simulink model "auditory_nerve_sim"  (R2020b)
settings: Solver=FixedStepDiscrete  StartTime=0.0  StopTime=stopTime  RelTol=1e-3
InitFcn:
  | initCallback
StopFcn:
  | stopCallback
values from neighbouring files (symbols this model uses):
  Fs = 48e3    (= 48000)    [modelparameters.m]
undefined symbols (not defined in the file or in its folder): mp
libraries: dspsrcs4 x1
settings Model: Creator=Ross  LastModifiedBy=wickh
settings DataIOCC: ReturnWorkspaceOutputs=off
settings OptimizationCC: BlockReduction=off  ConditionallyExecuteInputs=off  DefaultParameterBehavior=Inlined
settings DebuggingCC: ReadBeforeWriteMsg=DisableAll  WriteAfterWriteMsg=DisableAll  WriteAfterReadMsg=DisableAll  AlgebraicLoopMsg=error  MultiTaskDSMMsg=none  SingleTaskRateTransMsg=error  PregeneratedLibrarySubsystemCodeDiagnostic=none  ArithmeticOperatorsInVariantConditions=warning
settings HardwareCC: ProdBitPerPointer=32  ProdBitPerSizeT=32  ProdBitPerPtrDiffT=32  ProdLargestAtomicFloat=None  ProdIntDivRoundTo=Undefined  ProdEndianess=Unspecified  ProdWordSize=32  ProdHWDeviceType=ASIC/FPGA->ASIC/FPGA  TargetBitPerPointer=64  TargetBitPerSizeT=64  TargetBitPerPtrDiffT=64  TargetLongLongMode=on  TargetIntDivRoundTo=Zero  TargetEndianess=LittleEndian  TargetWordSize=64  TargetHWDeviceType=Custom Processor->MATLAB Host Computer  ProdEqTarget=off
settings ModelReferenceCC: UpdateModelReferenceTargets=IfOutOfDate
settings SFSimCC: SFSimEcho=off  SimUseLocalCustomCode=off  CustomCodeUndefinedFunction=UseInterfaceOnly
settings RTWCC: RTWUseLocalCustomCode=off

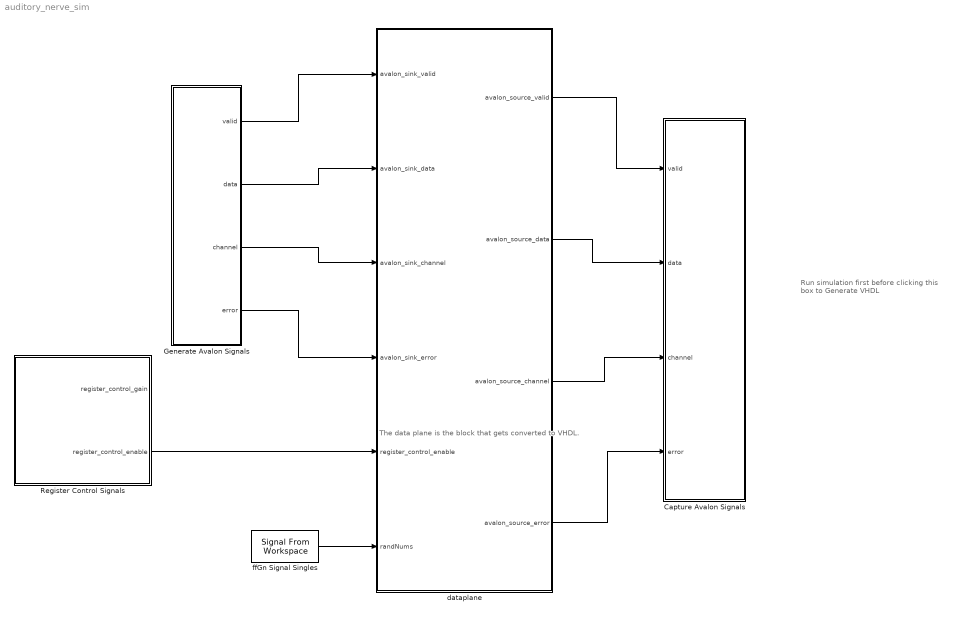
== system auditory_nerve_sim ==
  note: The data plane is the block that gets converted to VHDL.
  note: Run simulation first
      | before clicking this box to
      | Generate VHDL
  Capture Avalon Signals : Subsystem
  Generate Avalon Signals : Subsystem
  Register Control Signals : Subsystem
  dataplane : Subsystem  TreatAsAtomicUnit=on
  ffGn Signal Singles : dspsrcs4/Signal From Workspace  X=randNums  Ts=1/Fs  nsamps=1  OutputAfterFinalValue=Setting to zero  ignoreOrWarnInputAndFrameLengths=off  OutputFrames=off
  wires:
  Generate Avalon Signals/2(data) -> dataplane/2(avalon_sink_data)
  Generate Avalon Signals/1(valid) -> dataplane/1(avalon_sink_valid)
  Generate Avalon Signals/3(channel) -> dataplane/3(avalon_sink_channel)
  Generate Avalon Signals/4(error) -> dataplane/4(avalon_sink_error)
  dataplane/2(avalon_source_data) -> Capture Avalon Signals/2(data)
  dataplane/1(avalon_source_valid) -> Capture Avalon Signals/1(valid)
  dataplane/3(avalon_source_channel) -> Capture Avalon Signals/3(channel)
  dataplane/4(avalon_source_error) -> Capture Avalon Signals/4(error)
  Register Control Signals/2(register_control_enable) -> dataplane/5(register_control_enable)
  ffGn Signal Singles/1 -> dataplane/6(randNums)

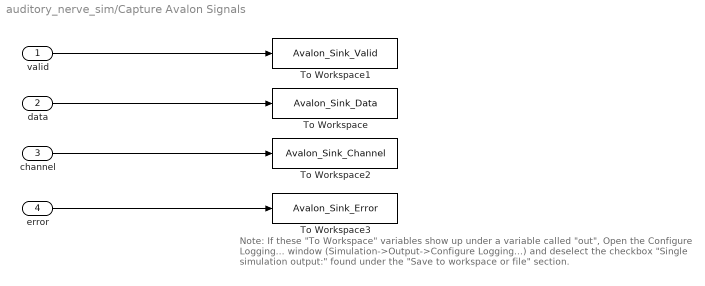
== system auditory_nerve_sim/Capture Avalon Signals ==
  note: Note:  If these "To Workspace" variables show up under a variable called "out",
      | Open the Configure Logging... window (Simulation->Output->Configure Logging...)
      | and deselect the checkbox "Single simulation output:" found under the "Save to workspace or file" section.
  valid : Inport
  data : Inport  Port=2
  channel : Inport  Port=3
  error : Inport  Port=4
  To Workspace : ToWorkspace  VariableName=Avalon_Sink_Data  SaveFormat=Timeseries  SampleTime=-1
  To Workspace1 : ToWorkspace  VariableName=Avalon_Sink_Valid  SaveFormat=Timeseries  SampleTime=-1
  To Workspace2 : ToWorkspace  VariableName=Avalon_Sink_Channel  SaveFormat=Timeseries  SampleTime=-1
  To Workspace3 : ToWorkspace  VariableName=Avalon_Sink_Error  SaveFormat=Timeseries  SampleTime=-1
  wires:
  data/1 -> To Workspace/1
  valid/1 -> To Workspace1/1
  error/1 -> To Workspace3/1
  channel/1 -> To Workspace2/1

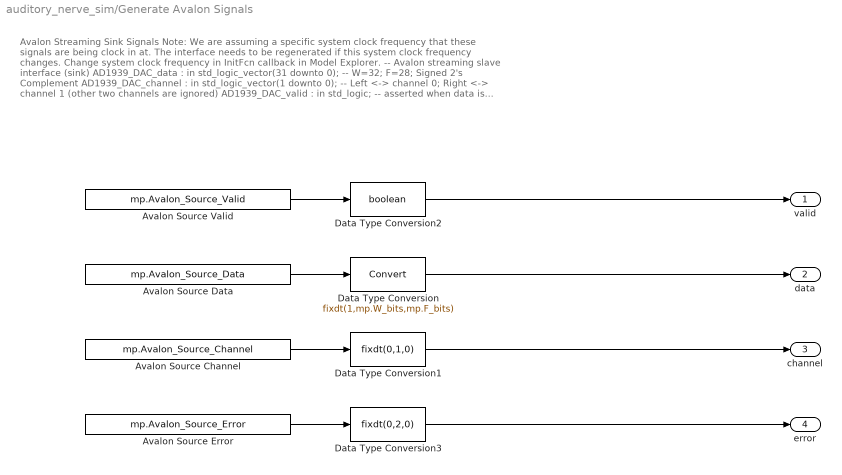
== system auditory_nerve_sim/Generate Avalon Signals ==
  note: Avalon Streaming Sink Signals
      | Note: We are assuming a specific system clock frequency that these signals are being clock in at.
      | The interface needs to be regenerated if this system clock frequency changes. Change system clock frequency in InitFcn callback in Model Explorer.
      |
      | -- Avalon streaming slave interface (sink)
      | AD1939_DAC_data : in std_logic_vector(31 downto 0); -- W=32; F=28; Signed 2's Complement
      | AD1939_DAC_channel : in std_logic_vector(1 downto 0); -- Left <-> channel 0; Right <-> channel 1 (other two channels are ignored)
      | AD1939_DAC_valid : in std_logic; -- asserted when data is valid
      | AD1939_DAC_error : in std_logic_vector(1 downto 0) -- error channel is ignored, assumed to be error free at this point
      |
      | For more information on the data-channel-valid protocol, s ee chapter 5 in Intel's Avalon Interfaced Specification (p. 40) at https://www.intel.com/content/dam/www/programmable/us/en/pdfs/literature/manual/mnl_avalon_spec.pdf
  Avalon Source Channel : FromWorkspace  VariableName=mp.Avalon_Source_Channel  OutDataTypeStr=double  SampleTime=mp.Ts_sim
  "Avalon Source Data " : FromWorkspace  VariableName=mp.Avalon_Source_Data  OutDataTypeStr=double  SampleTime=mp.Ts_sim
  Avalon Source Error : FromWorkspace  VariableName=mp.Avalon_Source_Error  OutDataTypeStr=double  SampleTime=mp.Ts_sim
  Avalon Source Valid : FromWorkspace  VariableName=mp.Avalon_Source_Valid  OutDataTypeStr=double  SampleTime=mp.Ts_sim
  Data Type Conversion : DataTypeConversion  OutDataTypeStr=fixdt(1,mp.W_bits,mp.F_bits)
  Data Type Conversion1 : DataTypeConversion  OutDataTypeStr=fixdt(0,1,0)
  Data Type Conversion2 : DataTypeConversion  OutDataTypeStr=boolean
  Data Type Conversion3 : DataTypeConversion  OutDataTypeStr=fixdt(0,2,0)
  valid : Outport  VectorParamsAs1DForOutWhenUnconnected=off
  data : Outport  Port=2  VectorParamsAs1DForOutWhenUnconnected=off
  channel : Outport  Port=3  VectorParamsAs1DForOutWhenUnconnected=off
  error : Outport  Port=4  VectorParamsAs1DForOutWhenUnconnected=off
  wires:
  Data Type Conversion1/1 -> channel/1
  Data Type Conversion2/1 -> valid/1
  Avalon Source Error/1 -> Data Type Conversion3/1
  Data Type Conversion/1 -> data/1
  Avalon Source Valid/1 -> Data Type Conversion2/1
  Data Type Conversion3/1 -> error/1
  Avalon Source Channel/1 -> Data Type Conversion1/1
  "Avalon Source Data "/1 -> Data Type Conversion/1

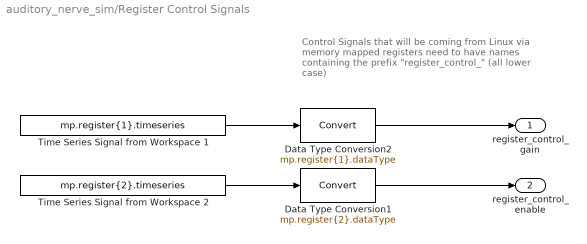
== system auditory_nerve_sim/Register Control Signals ==
  note: Control Signals that will be coming from Linux via
      | memory mapped registers need to have names
      | containing the prefix "register_control_"
      | (all lower case)
  Data Type Conversion1 : DataTypeConversion  OutDataTypeStr=mp.register{2}.dataType
  Data Type Conversion2 : DataTypeConversion  OutDataTypeStr=mp.register{1}.dataType
  Time Series Signal from Workspace 1 : FromWorkspace  VariableName=mp.register{1}.timeseries  OutDataTypeStr=double  SampleTime=mp.Ts_sim
  Time Series Signal from Workspace 2 : FromWorkspace  VariableName=mp.register{2}.timeseries  OutDataTypeStr=double  SampleTime=mp.Ts_sim
  register_control_gain : Outport  VectorParamsAs1DForOutWhenUnconnected=off
  register_control_enable : Outport  Port=2  VectorParamsAs1DForOutWhenUnconnected=off
  wires:
  Time Series Signal from Workspace 1/1 -> Data Type Conversion2/1
  Data Type Conversion2/1 -> register_control_gain/1
  Data Type Conversion1/1 -> register_control_enable/1
  Time Series Signal from Workspace 2/1 -> Data Type Conversion1/1

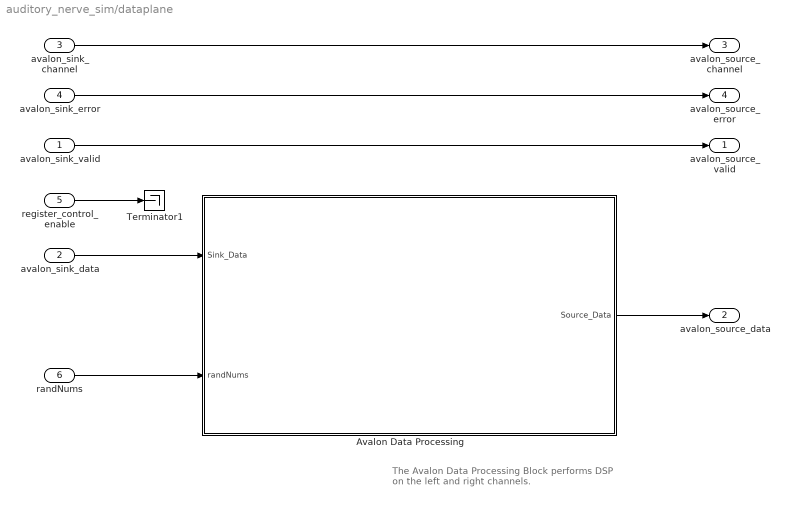
== system auditory_nerve_sim/dataplane ==
  note: The Avalon Data Processing Block
      | performs DSP on the left and right channels.
  avalon_sink_valid : Inport
  avalon_sink_data : Inport  Port=2
  avalon_sink_channel : Inport  Port=3
  avalon_sink_error : Inport  Port=4
  register_control_enable : Inport  Port=5
  randNums : Inport  Port=6
  Avalon Data Processing : Subsystem  TreatAsAtomicUnit=on
  Terminator1 : Terminator
  avalon_source_valid : Outport  VectorParamsAs1DForOutWhenUnconnected=off
  avalon_source_data : Outport  Port=2  VectorParamsAs1DForOutWhenUnconnected=off
  avalon_source_channel : Outport  Port=3  VectorParamsAs1DForOutWhenUnconnected=off
  avalon_source_error : Outport  Port=4  VectorParamsAs1DForOutWhenUnconnected=off
  wires:
  avalon_sink_error/1 -> avalon_source_error/1
  avalon_sink_valid/1 -> avalon_source_valid/1
  avalon_sink_data/1 -> Avalon Data Processing/1(Sink_Data)
  avalon_sink_channel/1 -> avalon_source_channel/1
  register_control_enable/1 -> Terminator1/1
  Avalon Data Processing/1(Source_Data) -> avalon_source_data/1
  randNums/1 -> Avalon Data Processing/2(randNums)

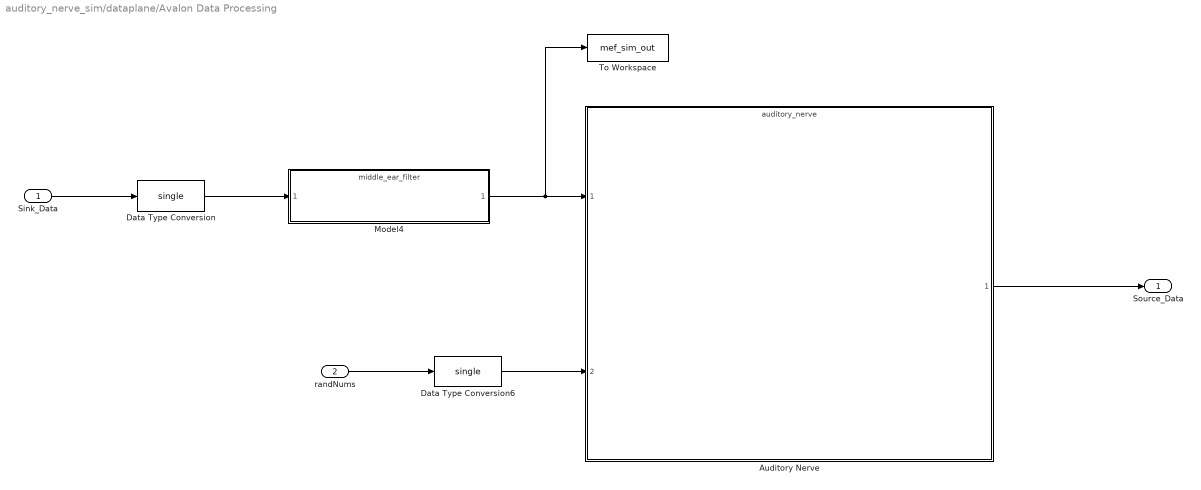
== system auditory_nerve_sim/dataplane/Avalon Data Processing ==
  Sink_Data : Inport
  randNums : Inport  Port=2
  Auditory Nerve : ModelReference  ModelNameDialog=auditory_nerve  SimulationMode=Normal  ModelReferenceVersion=1.153
  Data Type Conversion : DataTypeConversion  OutDataTypeStr=single
  Data Type Conversion6 : DataTypeConversion  OutDataTypeStr=single
  Model4 : ModelReference  ModelNameDialog=middle_ear_filter.slx  SimulationMode=Normal  ModelReferenceVersion=1.106
  To Workspace : ToWorkspace  VariableName=mef_sim_out  SaveFormat=Timeseries  SampleTime=-1
  Source_Data : Outport  InitialOutput=0  VectorParamsAs1DForOutWhenUnconnected=off
  wires:
  Sink_Data/1 -> Data Type Conversion/1
  Data Type Conversion6/1 -> Auditory Nerve/2
  randNums/1 -> Data Type Conversion6/1
  Auditory Nerve/1 -> Source_Data/1
  Data Type Conversion/1 -> Model4/1
  Model4/1 -> To Workspace/1, Auditory Nerve/1
